simulink model "converterControltest"  (R2023b)
settings: Solver=VariableStepAuto  StartTime=0.0  StopTime=10.0  RelTol=1e-3
undefined symbols (not defined in the file): Ibase_lv, Ki_cc, Ki_vc, Kp_cc, Kp_vc, L_f, l_f, omega_nom, R_f, r_f, Sbase1, Vbase_lv
libraries: spsControlledVoltageSourceLib x3, spsMultimeterLib x2, spsSequenceAnalyzerLib x2, spsabctodq0Lib x2, spsGroundLib x1, spsThreePhaseSeriesRLCBranchLib x1, spsThreePhaseVIMeasurementLib x1, spsThreePhaseSourceLib x1, spsdq0toabcLib x1, sps_lib x1, spsPower3phInstantaneousLib x1
settings Model: Creator=s183702  LastModifiedBy=marti

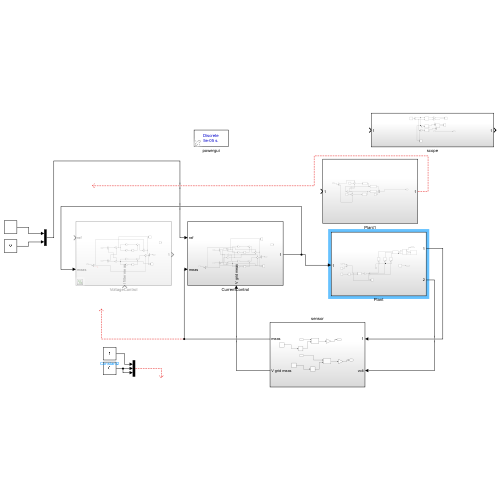
[thumbnail: Simulink's stored preview of the top-level diagram]
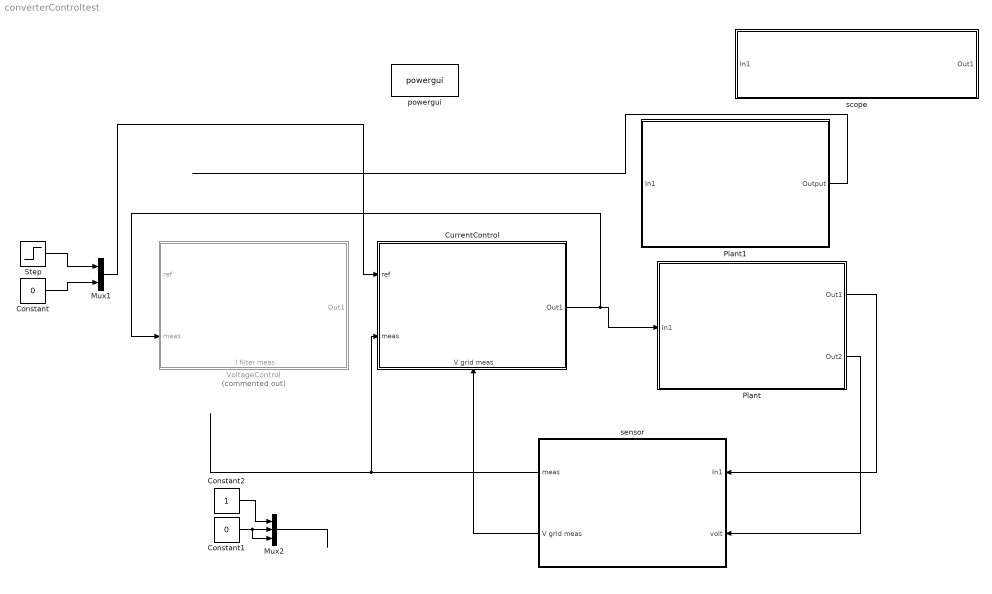
== system converterControltest ==
  Constant : Constant  Value=0
  Constant1 : Constant  Value=0
  Constant2 : Constant
  CurrentControl : Subsystem
      settings: PortSchema="{\"entries\":[{\"content\":{\"sides\":[{\"content\":{\"connectorIds\":[\"In1\",\"In2\"]},\"type\":\"ConnectorPlacement.EquallySpacedRectSide\",\"uuid\":\"219db9ea-637c-42c0-b87e-0a8373949a2f\"},{\"content\":{\"connectorIds\":[\"Out1\"],\"side\":\"RIGHT\"},\"type\":\"ConnectorPlacement.EquallySpacedRectSide\",\"uuid\":\"817edf77-a627-4761-8536-4c41ccdce557\"},{\"content\":{\"side\":\"TOP\"},\"type\":\"ConnectorPlacement.EquallySpacedRectSide\",\"uuid\":\"b4d64eff-9104-48e3-a4e2-ec81b224adc3\"},{\"content\":{\"connectorIds\":[\"In3\"],\"side\":\"BOTTOM\"},\"type\":\"ConnectorPlacement.EquallySpacedRectSide\",\"uuid\":\"8db682a6-86bb-4d51-9cc3-8f643a502240\"}]},\"type\":\"ConnectorPlacement.EquallySpacedConnector\",\"uuid\":\"cfbf309f-cee6-401c-8c28-748b4359d9c9\"}],\"packageUris\":[\"http://schema.mathworks.com/mf0/Connector/R2020b\"],\"version\":\"1.0\"}"
  Mux1 : Mux  Inputs=2
  Mux2 : Mux  Inputs=3
  Plant : Subsystem
  Plant1 : Subsystem
  Step : Step  Time=5  Before=1  After=2  SampleTime=0
  VoltageControl : Subsystem  Commented=on
      settings: PortSchema="{\"entries\":[{\"content\":{\"sides\":[{\"content\":{\"connectorIds\":[\"In1\",\"In2\"]},\"type\":\"ConnectorPlacement.EquallySpacedRectSide\",\"uuid\":\"219db9ea-637c-42c0-b87e-0a8373949a2f\"},{\"content\":{\"connectorIds\":[\"Out1\"],\"side\":\"RIGHT\"},\"type\":\"ConnectorPlacement.EquallySpacedRectSide\",\"uuid\":\"817edf77-a627-4761-8536-4c41ccdce557\"},{\"content\":{\"side\":\"TOP\"},\"type\":\"ConnectorPlacement.EquallySpacedRectSide\",\"uuid\":\"b4d64eff-9104-48e3-a4e2-ec81b224adc3\"},{\"content\":{\"connectorIds\":[\"In3\"],\"side\":\"BOTTOM\"},\"type\":\"ConnectorPlacement.EquallySpacedRectSide\",\"uuid\":\"8db682a6-86bb-4d51-9cc3-8f643a502240\"}]},\"type\":\"ConnectorPlacement.EquallySpacedConnector\",\"uuid\":\"cfbf309f-cee6-401c-8c28-748b4359d9c9\"}],\"packageUris\":[\"http://schema.mathworks.com/mf0/Connector/R2020b\"],\"version\":\"1.0\"}"
  powergui : sps_lib/powergui  Priority=1  SimulationMode=Discrete  SampleTime=50e-6  frequency=60  Iterations=50  frequencyindice=50  Pbase=100e6  ErrMax=1e-4  UnitsV=kV  UnitsW=MW  buscounter=0  FunctionMessages=off  echomessages=off  EnableUseOfTLC=off  CurrentSourceSwitches=off  DisableSnubberDevices=off  DisableRonSwitches=off  DisableVfSwitches=off  DisplayEquations=off  AutomaticDiscreteSolvers=off  SolverType=Tustin/Backward Euler (TBE)  Interpol=off  ExternalGateDelay=off  methode=off  Ts=100  x0status=blocks  SPID=on  SwTol=0  HookPort=off  NonlinearTolerance=1e-4  nMaxIteration=100  ContinueOnMaxIteration=off  RestoreLinks=warning  ResistiveCurrentMeasurement=off  Frange=[0:2:500]  Ylog=off  Xlog=on  ShowGrid=off  save=off  variable=ZData  structure=0  ZoomFFT=off  StartTime=0.0  cycles=1  DisplayStyle=1  fundamental=60  FreqAxis=off  MaxFrequency=1000  frequencyindicesteady=1  RmsSteady=1  display=off
  scope : Subsystem
  sensor : Subsystem
  wires:
  Plant/1(Out1) -> sensor/1(In1)
  sensor/1(meas) -> CurrentControl/2(meas)
  Constant/1 -> Mux1/2
  Step/1 -> Mux1/1
  CurrentControl/1(Out1) -> VoltageControl/2(meas), Plant/1(In1)
  Plant/2(Out2) -> sensor/2(volt)
  sensor/2(V grid meas) -> CurrentControl/3(V grid meas)
  Plant1/1(Output) -> ?
  Constant1/1 -> Mux2/3, Mux2/2
  Constant2/1 -> Mux2/1
  Mux2/1 -> ?
  Mux1/1 -> CurrentControl/1(ref)

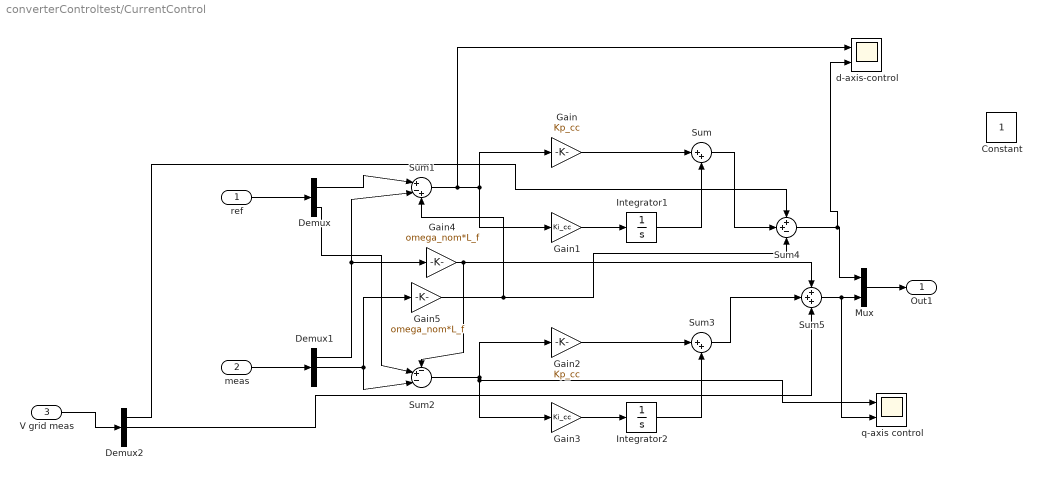
== system converterControltest/CurrentControl ==
  ref : Inport
  meas : Inport  Port=2
  V grid meas : Inport  Port=3
  Constant : Constant
  Demux : Demux  Outputs=2
  Demux1 : Demux  Outputs=3
  Demux2 : Demux  Outputs=3
  Gain : Gain  Gain=Kp_cc
  Gain1 : Gain  Gain=Ki_cc
  Gain2 : Gain  Gain=Kp_cc
  Gain3 : Gain  Gain=Ki_cc
  Gain4 : Gain  Gain=omega_nom*L_f
  Gain5 : Gain  Gain=omega_nom*L_f
  Integrator1 : Integrator
  Integrator2 : Integrator
  Mux : Mux  Inputs=2
  Sum : Sum  Inputs=|++
  Sum1 : Sum  Inputs=|+-+
  Sum2 : Sum  Inputs=-+-|
  Sum3 : Sum  Inputs=|++
  Sum4 : Sum  Inputs=++-
  Sum5 : Sum  Inputs=+++
  d-axis-control : Scope  NumInputPorts=2
  q-axis control : Scope  NumInputPorts=2
  Out1 : Outport
  wires:
  Mux/1 -> Out1/1
  Gain/1 -> Sum/1
  Integrator1/1 -> Sum/2
  Gain1/1 -> Integrator1/1
  Sum1/1 -> d-axis-control/1, Gain1/1, Gain/1
  ref/1 -> Demux/1
  meas/1 -> Demux1/1
  Demux1/2 -> Sum2/3, Gain5/1
  Demux1/1 -> Gain4/1, Sum1/2
  Demux/2 -> Sum2/2
  Demux/1 -> Sum1/1
  Sum/1 -> Sum4/2
  Sum3/1 -> Sum5/2
  Gain3/1 -> Integrator2/1
  Integrator2/1 -> Sum3/2
  Gain2/1 -> Sum3/1
  Sum2/1 -> q-axis control/1, Gain3/1, Gain2/1
  Sum4/1 -> d-axis-control/2, Mux/1
  Gain5/1 -> Sum4/3, Sum1/3
  Gain4/1 -> Sum2/1, Sum5/1
  Demux2/2 -> Sum5/3
  Sum5/1 -> q-axis control/2, Mux/2
  V grid meas/1 -> Demux2/1
  Demux2/1 -> Sum4/1

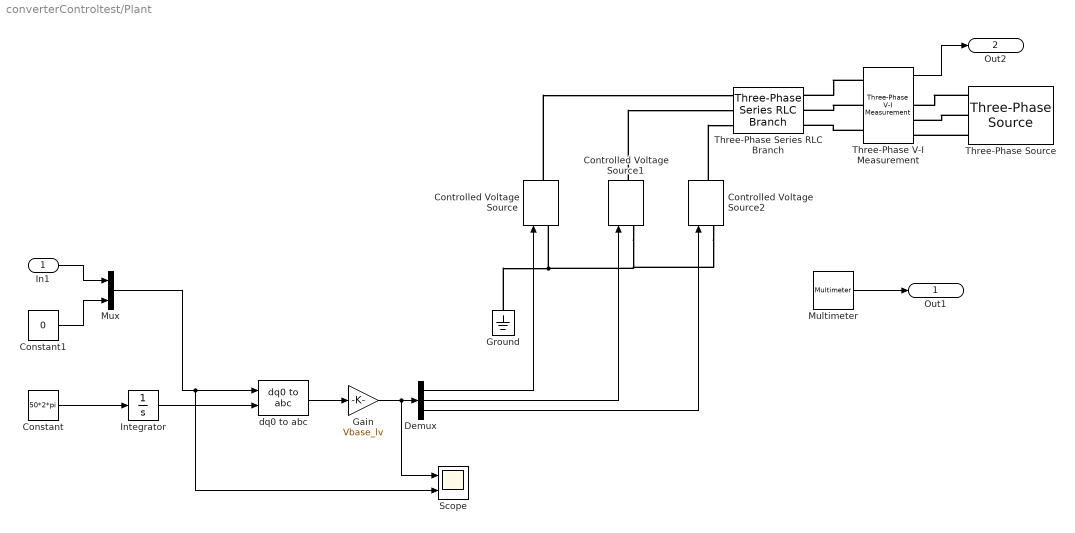
== system converterControltest/Plant ==
  In1 : Inport
  Constant : Constant  Value=50*2*pi
  Constant1 : Constant  Value=0
  Controlled Voltage Source : spsControlledVoltageSourceLib/Controlled Voltage Source  Initialize=on  Source_Type=AC  Amplitude=0  Phase=0  Frequency=0  Measurements=Voltage
  Controlled Voltage Source1 : spsControlledVoltageSourceLib/Controlled Voltage Source  Initialize=on  Source_Type=AC  Amplitude=0  Phase=0  Frequency=0  Measurements=Voltage
  Controlled Voltage Source2 : spsControlledVoltageSourceLib/Controlled Voltage Source  Initialize=on  Source_Type=AC  Amplitude=0  Phase=0  Frequency=0  Measurements=Voltage
  Demux : Demux  Outputs=3
  Gain : Gain  Gain=Vbase_lv
  Ground : spsGroundLib/Ground  LConnTagsString=a
  Integrator : Integrator
  Multimeter : spsMultimeterLib/Multimeter  L=6  sel=[4 5 6]  yselected={}  Gain=[1 1 1]  OutputType=Complex  PlotAtSimulationStop=off  PhasorSimulation=off
  Mux : Mux  Inputs=2
  Scope : Scope  NumInputPorts=2
  Three-Phase Series RLC Branch : spsThreePhaseSeriesRLCBranchLib/Three-Phase Series RLC Branch  LConnTagsString=A|B|C  RConnTagsString=A|B|C  BranchType=RL  Resistance=R_f  Inductance=L_f  Capacitance=1e-6  Measurements=Branch currents
  Three-Phase V-I Measurement : spsThreePhaseVIMeasurementLib/Three-Phase V-I Measurement  VoltageMeasurement=phase-to-ground  SetLabelV=off  LabelV=Vabc  Vpu=off  VpuLL=off  CurrentMeasurement=yes  SetLabelI=off  LabelI=Iabc  Ipu=off  Pbase=100e6  Vbase=500e3  OutputType=Complex  PhasorSimulation=off  PSBequivalent=0
  Three-Phase Source : spsThreePhaseSourceLib/Three-Phase Source  InternalConnection=Yg  VoltagePhases=off  Voltage=Vbase_lv*sqrt(3)/sqrt(2)  PhaseAngle=0  Voltage_phases=[25e3 25e3 25e3]/sqrt(3)  PhaseAngles_phases=[0 -120 +120]  Frequency=50  NonIdealSource=off  SpecifyImpedance=off  Resistance=0.8929  Inductance=16.58e-3  ShortCircuitLevel=100e6  BaseVoltage=25e3  XRratio=7  BusType=swing  Pref=10e3  Qref=0  Prefabc=[10e3, 10e3, 10e3]  Qrefabc=[0, 0, 0]  Qmin=-inf  Qmax=inf
  dq0 to abc : spsdq0toabcLib/dq0 to abc  Alignment=90 degrees behind phase A axis
  Out1 : Outport
  Out2 : Outport  Port=2
  wires:
  Mux/1 -> Scope/2, dq0 to abc/1
  Demux/1 -> Controlled Voltage Source/1
  Demux/2 -> Controlled Voltage Source1/1
  Demux/3 -> Controlled Voltage Source2/1
  dq0 to abc/1 -> Gain/1
  Constant/1 -> Integrator/1
  Multimeter/1 -> Out1/1
  Integrator/1 -> dq0 to abc/2
  Constant1/1 -> Mux/2
  In1/1 -> Mux/1
  Gain/1 -> Scope/1, Demux/1
  Three-Phase V-I Measurement/1 -> Out2/1
  connections:
  Ground/LConn1 -- Controlled Voltage Source2/LConn1 -- Controlled Voltage Source1/LConn1 -- Controlled Voltage Source/LConn1
  Controlled Voltage Source2/RConn1 -- Three-Phase Series RLC Branch/LConn3
  Controlled Voltage Source1/RConn1 -- Three-Phase Series RLC Branch/LConn2
  Controlled Voltage Source/RConn1 -- Three-Phase Series RLC Branch/LConn1
  Three-Phase Source/RConn1 -- Three-Phase V-I Measurement/RConn1
  Three-Phase Source/RConn2 -- Three-Phase V-I Measurement/RConn2
  Three-Phase Source/RConn3 -- Three-Phase V-I Measurement/RConn3
  Three-Phase V-I Measurement/LConn1 -- Three-Phase Series RLC Branch/RConn1
  Three-Phase V-I Measurement/LConn2 -- Three-Phase Series RLC Branch/RConn2
  Three-Phase V-I Measurement/LConn3 -- Three-Phase Series RLC Branch/RConn3

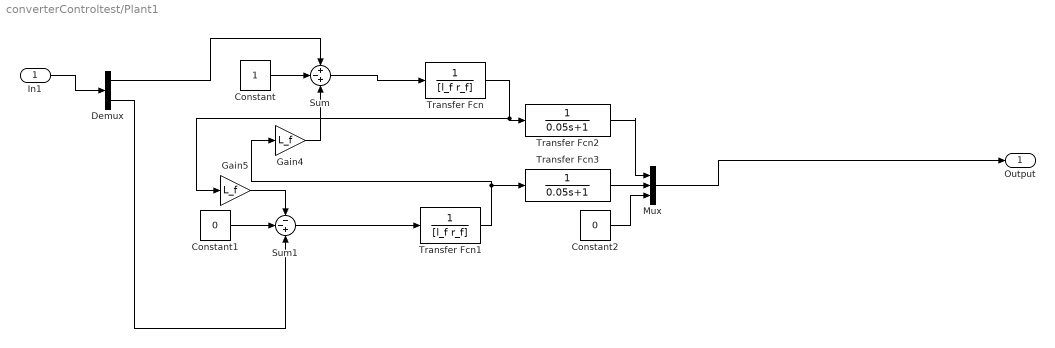
== system converterControltest/Plant1 ==
  In1 : Inport
  Constant : Constant
  Constant1 : Constant  Value=0
  Constant2 : Constant  Value=0
  Demux : Demux  Outputs=2
  Gain4 : Gain  Gain=L_f
  Gain5 : Gain  Gain=L_f
  Mux : Mux  Inputs=3
  Sum : Sum  Inputs=+-+
  Sum1 : Sum  Inputs=--+
  Transfer Fcn : TransferFcn  Denominator=[l_f r_f]
  Transfer Fcn1 : TransferFcn  Denominator=[l_f r_f]
  Transfer Fcn2 : TransferFcn  Denominator=[0.05 1]
  Transfer Fcn3 : TransferFcn  Denominator=[0.05 1]
  Output : Outport
  wires:
  In1/1 -> Demux/1
  Gain4/1 -> Sum/3
  Gain5/1 -> Sum1/1
  Transfer Fcn/1 -> Transfer Fcn2/1, Gain5/1
  Transfer Fcn1/1 -> Transfer Fcn3/1, Gain4/1
  Demux/1 -> Sum/1
  Constant/1 -> Sum/2
  Constant1/1 -> Sum1/2
  Demux/2 -> Sum1/3
  Sum/1 -> Transfer Fcn/1
  Sum1/1 -> Transfer Fcn1/1
  Constant2/1 -> Mux/3
  Mux/1 -> Output/1
  Transfer Fcn2/1 -> Mux/1
  Transfer Fcn3/1 -> Mux/2

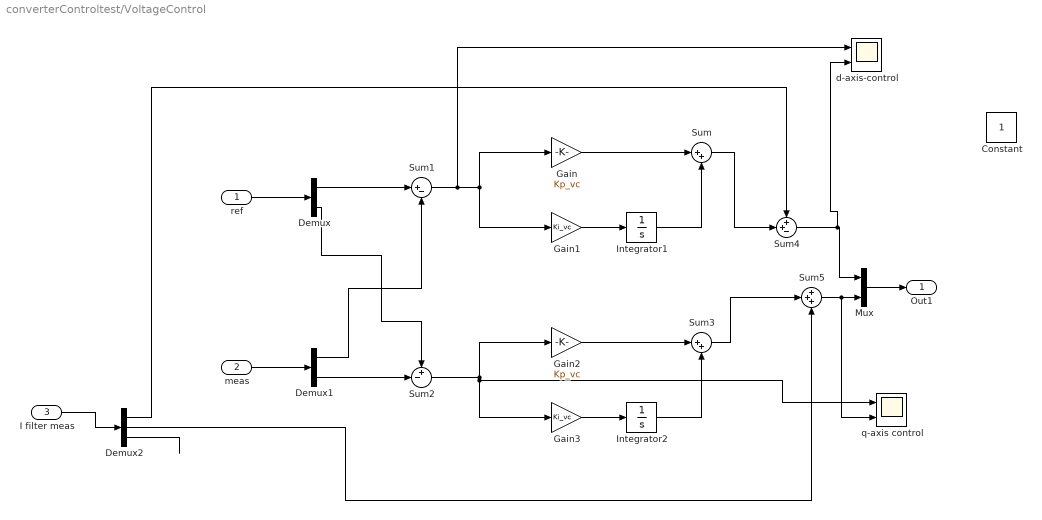
== system converterControltest/VoltageControl ==
  ref : Inport
  meas : Inport  Port=2
  I filter meas : Inport  Port=3
  Constant : Constant
  Demux : Demux  Outputs=2
  Demux1 : Demux  Outputs=2
  Demux2 : Demux  Outputs=3
  Gain : Gain  Gain=Kp_vc
  Gain1 : Gain  Gain=Ki_vc
  Gain2 : Gain  Gain=Kp_vc
  Gain3 : Gain  Gain=Ki_vc
  Integrator1 : Integrator
  Integrator2 : Integrator
  Mux : Mux  Inputs=2
  Sum : Sum  Inputs=|++
  Sum1 : Sum  Inputs=|+-
  Sum2 : Sum  Inputs=+-|
  Sum3 : Sum  Inputs=|++
  Sum4 : Sum  Inputs=++-
  Sum5 : Sum  Inputs=+++
  d-axis-control : Scope  NumInputPorts=2
  q-axis control : Scope  NumInputPorts=2
  Out1 : Outport
  wires:
  Demux2/1 -> Sum4/1
  I filter meas/1 -> Demux2/1
  Sum5/1 -> Mux/2, q-axis control/2
  Demux2/2 -> Sum5/3
  Sum4/1 -> Mux/1, d-axis-control/2
  Sum2/1 -> Gain2/1, Gain3/1, q-axis control/1
  Gain2/1 -> Sum3/1
  Integrator2/1 -> Sum3/2
  Gain3/1 -> Integrator2/1
  Sum3/1 -> Sum5/2
  Sum/1 -> Sum4/2
  Demux/1 -> Sum1/1
  Demux/2 -> Sum2/1
  Demux1/1 -> Sum1/2
  Demux1/2 -> Sum2/2
  meas/1 -> Demux1/1
  ref/1 -> Demux/1
  Sum1/1 -> Gain/1, Gain1/1, d-axis-control/1
  Gain1/1 -> Integrator1/1
  Integrator1/1 -> Sum/2
  Gain/1 -> Sum/1
  Mux/1 -> Out1/1
  Demux2/3 -> ?

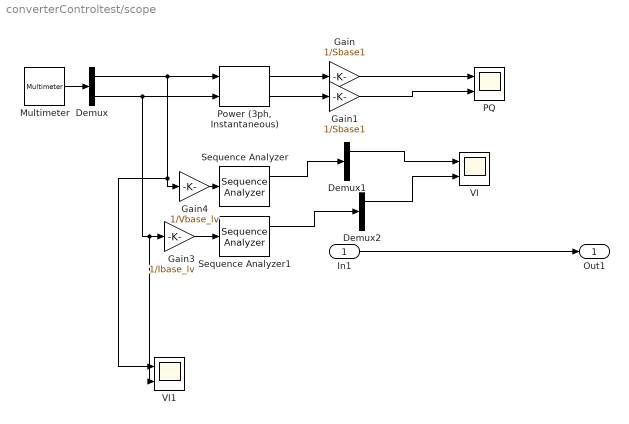
== system converterControltest/scope ==
  In1 : Inport
  Demux : Demux  Outputs=2
  Demux1 : Demux  Outputs=3
  Demux2 : Demux  Outputs=3
  Gain : Gain  Gain=1/Sbase1
  Gain1 : Gain  Gain=1/Sbase1
  Gain3 : Gain  Gain=1/Ibase_lv
  Gain4 : Gain  Gain=1/Vbase_lv
  Multimeter : spsMultimeterLib/Multimeter  L=6  sel=[1 2 3 4 5 6]  yselected={}  Gain=[1 1 1 1 1 1]  OutputType=Complex  PlotAtSimulationStop=off  PhasorSimulation=off
  PQ : Scope  NumInputPorts=2
  "Power (3ph, Instantaneous)" : spsPower3phInstantaneousLib/Power (3ph, Instantaneous)
  Sequence Analyzer : spsSequenceAnalyzerLib/Sequence Analyzer  Freq=60  n=1  seq=Positive Negative Zero  InInit=[1, 0]  Ts=0
      settings: LibrarySourceBlock=sps_lib/Sensors and Measurements/Sequence Analyzer
  Sequence Analyzer1 : spsSequenceAnalyzerLib/Sequence Analyzer  Freq=60  n=1  seq=Positive Negative Zero  InInit=[1, 0]  Ts=0
      settings: LibrarySourceBlock=sps_lib/Sensors and Measurements/Sequence Analyzer
  VI : Scope  NumInputPorts=2
  VI1 : Scope  NumInputPorts=2
  Out1 : Outport
  wires:
  In1/1 -> Out1/1
  Multimeter/1 -> Demux/1
  "Power (3ph, Instantaneous)"/1 -> Gain/1
  "Power (3ph, Instantaneous)"/2 -> Gain1/1
  Gain/1 -> PQ/1
  Gain1/1 -> PQ/2
  Demux/1 -> VI1/1, Gain4/1, "Power (3ph, Instantaneous)"/1
  Demux/2 -> VI1/2, Gain3/1, "Power (3ph, Instantaneous)"/2
  Sequence Analyzer/1 -> Demux1/1
  Gain3/1 -> Sequence Analyzer1/1
  Gain4/1 -> Sequence Analyzer/1
  Demux1/1 -> VI/1
  Demux2/1 -> VI/2
  Sequence Analyzer1/1 -> Demux2/1

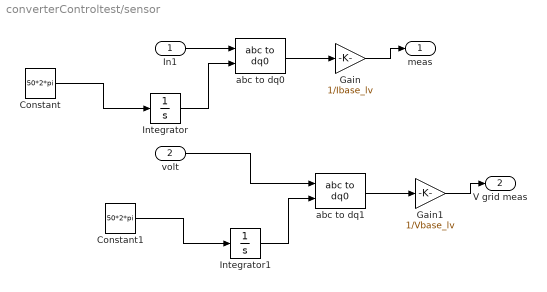
== system converterControltest/sensor ==
  In1 : Inport
  volt : Inport  Port=2
  Constant : Constant  Value=50*2*pi
  Constant1 : Constant  Value=50*2*pi
  Gain : Gain  Gain=1/Ibase_lv
  Gain1 : Gain  Gain=1/Vbase_lv
  Integrator : Integrator
  Integrator1 : Integrator
  abc to dq0 : spsabctodq0Lib/abc to dq0  Alignment=90 degrees behind phase A axis
  abc to dq1 : spsabctodq0Lib/abc to dq0  Alignment=90 degrees behind phase A axis
  meas : Outport
  V grid meas : Outport  Port=2
  wires:
  In1/1 -> abc to dq0/1
  Constant/1 -> Integrator/1
  Integrator/1 -> abc to dq0/2
  abc to dq0/1 -> Gain/1
  Gain/1 -> meas/1
  Gain1/1 -> V grid meas/1
  abc to dq1/1 -> Gain1/1
  Integrator1/1 -> abc to dq1/2
  Constant1/1 -> Integrator1/1
  volt/1 -> abc to dq1/1
